simulink model "slewmode"  (R2024a)
settings: Solver=ode45  StartTime=0.0  StopTime=2000  MaxStep=20  RelTol=1e-6  EnableMultiTasking=on
values from neighbouring files (symbols this model uses):
  I = [3000 0 0 ... (first row only)    [Constants_gui.m]    (also in constants.m; mbi.m = [15, .25, .20; set_up_HW7.m = I-Id; setupConstantRateSDA.m)
  invI = inv(I)    [Constants_gui.m]    (also in constants.m; mbi.m; set_up_HW7.m; setupConstantRateSDA.m)
  Kd = 2*zet*wn*I    [Constants_gui.m]    (also in constants.m = 2 * zet * wn * I; mbi.m = -eye(3)*.00002; set_up_HW7.m = 375000; setupConstantRateSDA.m)
  Kp = 2*wn^2*I    [Constants_gui.m]    (also in constants.m = 2 * wn^2 * I; mbi.m = -eye(3)*5.5; set_up_HW7.m = 300000; setupConstantRateSDA.m)
  q_c = q_c / norm(q_c)    [constants.m]
  q_init = q_init/norm(q_init)    [Constants_gui.m]    (also in constants.m = [-0.5 -0.5 -0.5 0.5]; mbi.m = [0 0 0 1]'; set_up_HW7.m = [0 0 0 1]'; setupConstantRateSDA.m)
  wbn_init = pi/30*[0 0 0]'    [Constants_gui.m]    (also in constants.m = pi/180 * [0.1; 0.2; 0.15]; mbi.m = [0 0 0]'; set_up_HW7.m = pi/30*[0 0 .01]'; setupConstantRateSDA.m)
libraries: aerolibutil x2
settings Model: Creator=Mason  LastModifiedBy=robertbergbaum
settings SolverCC: AlgebraicLoopSolver=TrustRegion  MaxZcPerStep=1
settings DataIOCC: LimitDataPoints=on  SaveFormat=Array  SignalLoggingSaveFormat=ModelDataLogs  ReturnWorkspaceOutputs=off
settings OptimizationCC: ExpressionDepthLimit=2147483647  InitFltsAndDblsToZero=on  LifeSpan=inf
settings DebuggingCC: SaveWithParameterizedLinksMsg=none  UnderspecifiedInitializationDetection=Classic  MergeDetectMultiDrivingBlocksExec=none  SignalResolutionControl=TryResolveAllWithWarning  SolverPrmCheckMsg=warning  MultiTaskDSMMsg=warning  MultiTaskCondExecSysMsg=none  FcnCallInpInsideContextMsg=warning  UnconnectedInputMsg=warning  UnconnectedOutputMsg=warning  UnconnectedLineMsg=warning  StateNameClashWarn=warning  SFUnexpectedBacktrackingDiag=warning  SFNoUnconditionalDefaultTransitionDiag=warning  SFExecutionAtInitializationDiag=none  ArithmeticOperatorsInVariantConditions=warning
settings HardwareCC: ProdBitPerPointer=32  ProdBitPerSizeT=32  ProdBitPerPtrDiffT=32  ProdLargestAtomicFloat=None  ProdIntDivRoundTo=Undefined  ProdEndianess=Unspecified  ProdWordSize=32  ProdHWDeviceType=32-bit Generic
settings ModelReferenceCC: EnableRefExpFcnMdlSchedulingChecks=on  PropagateSignalLabelsOutOfModel=off
settings SFSimCC: SimUseLocalCustomCode=off  CustomCodeUndefinedFunction=UseInterfaceOnly
settings RTWCC: RTWUseLocalCustomCode=off  GPUComputeCapability=3.5  DLArmComputeVersion=19.05
settings CodeAppCC: StateflowObjectComments=on
settings GRTTargetCC: TargetFcnLib=ansi_tfl_tmw.mat  TargetLangStandard=C89/C90 (ANSI)  CombineOutputUpdateFcns=off  GRTInterface=on
settings ConfigComp: CovMetricSettings=dw  CovSaveCumulativeToWorkspaceVar=on  CovSaveSingleToWorkspaceVar=on  CovExternalEMLEnable=off

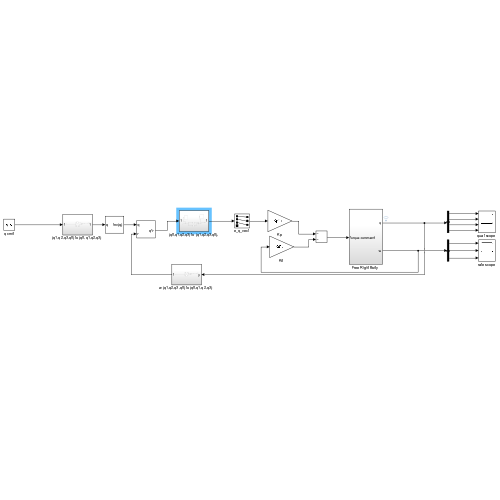
[thumbnail: Simulink's stored preview of the top-level diagram]
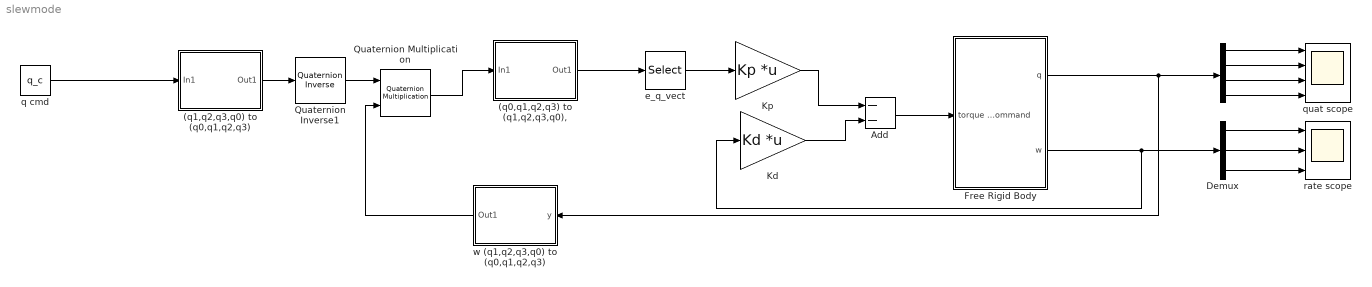
== system slewmode ==
  " " : Demux
      settings: DisplayOption=none
  (q0,q1,q2,q3) to (q1,q2,q3,q0), : Subsystem
  "(q1,q2,q3,q0) to (q0,q1,q2,q3) " : Subsystem
  Add : Sum  Inputs=--
  Demux : Demux  Outputs=3
      settings: DisplayOption=none
  "Free Rigid Body " : Subsystem
  Kd : Gain  Gain=Kd  Multiplication=Matrix(K*u)  SaturateOnIntegerOverflow=on  OutDataTypeStr=Inherit: Same as input  ParamDataTypeStr=Inherit: Same as input
  Kp : Gain  Gain=Kp  Multiplication=Matrix(K*u)  SaturateOnIntegerOverflow=on  OutDataTypeStr=Inherit: Same as input  ParamDataTypeStr=Inherit: Same as input
  Quaternion Inverse1 : aerolibutil/Quaternion Inverse
  Quaternion Multiplication : aerolibutil/Quaternion Multiplication
  e_q_vect : Selector  InputPortWidth=4  IndexOptions=Index vector (dialog)  Indices=[1 2 3]  OutputSizes=1
  q cmd : Constant  Value=q_c  VectorParams1D=off
  quat scope : Scope  NumInputPorts=4
  rate scope : Scope  NumInputPorts=3
  "w (q1,q2,q3,q0) to (q0,q1,q2,q3) " : Subsystem
      settings: PortSchema="{\"entries\":[{\"content\":{\"sides\":[{\"content\":{\"connectorIds\":[\"Out1\"]},\"type\":\"ConnectorPlacement.EquallySpacedRectSide\",\"uuid\":\"97b477ad-5663-4010-b344-d27b8ec095be\"},{\"content\":{\"connectorIds\":[\"In1\"],\"side\":\"RIGHT\"},\"type\":\"ConnectorPlacement.EquallySpacedRectSide\",\"uuid\":\"41fe4029-0263-4427-bdfc-3c26258b8a65\"},{\"content\":{\"side\":\"TOP\"},\"type\":\"ConnectorPlacement.EquallySpacedRectSide\",\"uuid\":\"9fb3a03d-539a-4245-bd7d-8174d3d0797f\"}]},\"type\":\"ConnectorPlacement.EquallySpacedConnector\",\"uuid\":\"44222554-f3ae-4bc6-b92c-7571a5ce84f7\"}],\"packageUris\":[\"http://schema.mathworks.com/mf0/Connector/R2020b\"],\"version\":\"1.0\"}"
  wires:
  Kd/1 -> Add/2
  Demux/2 -> rate scope/2
  Demux/3 -> rate scope/3
  Demux/1 -> rate scope/1
  "Free Rigid Body "/2(w) -> Kd/1, Demux/1
  " "/1 -> quat scope/1
  " "/2 -> quat scope/2
  " "/3 -> quat scope/3
  " "/4 -> quat scope/4
  e_q_vect/1 -> Kp/1
  "Free Rigid Body "/1(q) -> "w (q1,q2,q3,q0) to (q0,q1,q2,q3) "/1(y), " "/1
  Kp/1 -> Add/1
  Add/1 -> "Free Rigid Body "/1(torque command)
  Quaternion Multiplication/1 -> (q0,q1,q2,q3) to (q1,q2,q3,q0),/1(In1)
  (q0,q1,q2,q3) to (q1,q2,q3,q0),/1(Out1) -> e_q_vect/1
  "(q1,q2,q3,q0) to (q0,q1,q2,q3) "/1(Out1) -> Quaternion Inverse1/1
  "w (q1,q2,q3,q0) to (q0,q1,q2,q3) "/1(Out1) -> Quaternion Multiplication/2
  Quaternion Inverse1/1 -> Quaternion Multiplication/1
  q cmd/1 -> "(q1,q2,q3,q0) to (q0,q1,q2,q3) "/1(In1)

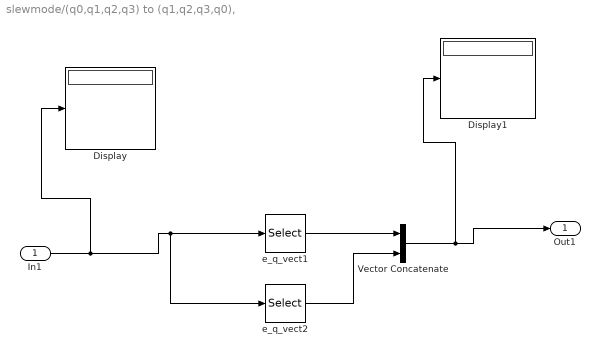
== system slewmode/(q0,q1,q2,q3) to (q1,q2,q3,q0), ==
  In1 : Inport
  Display : Display
  Display1 : Display
  Vector Concatenate : Concatenate
  e_q_vect1 : Selector  InputPortWidth=4  IndexOptions=Index vector (dialog)  Indices=[2 3 4]  OutputSizes=1
  e_q_vect2 : Selector  InputPortWidth=4  IndexOptions=Index vector (dialog)  Indices=[1]  OutputSizes=1
  Out1 : Outport
  wires:
  Vector Concatenate/1 -> Display1/1, Out1/1
  In1/1 -> Display/1, e_q_vect2/1, e_q_vect1/1
  e_q_vect1/1 -> Vector Concatenate/1
  e_q_vect2/1 -> Vector Concatenate/2

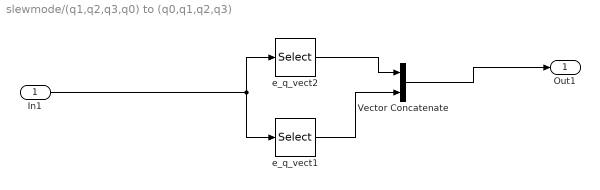
== system slewmode/(q1,q2,q3,q0) to (q0,q1,q2,q3)  ==
  In1 : Inport
  Vector Concatenate : Concatenate
  e_q_vect1 : Selector  InputPortWidth=4  IndexOptions=Index vector (dialog)  Indices=[1 2 3]  OutputSizes=1
  e_q_vect2 : Selector  InputPortWidth=4  IndexOptions=Index vector (dialog)  Indices=[4]  OutputSizes=1
  Out1 : Outport
  wires:
  In1/1 -> e_q_vect2/1, e_q_vect1/1
  e_q_vect2/1 -> Vector Concatenate/1
  e_q_vect1/1 -> Vector Concatenate/2
  Vector Concatenate/1 -> Out1/1

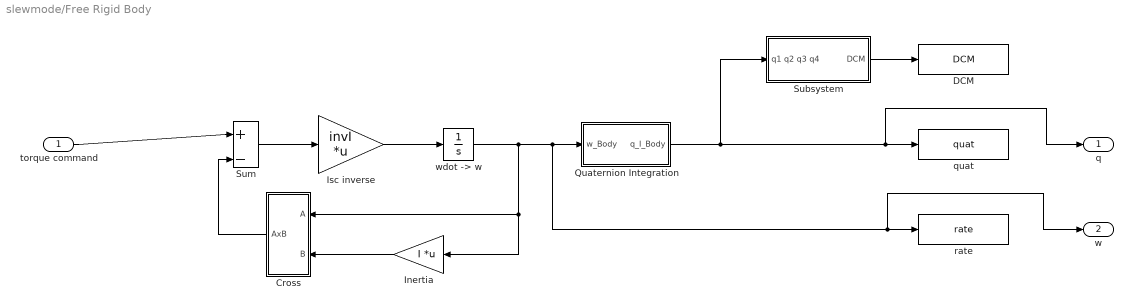
== system slewmode/Free Rigid Body  ==
  torque command : Inport
  Cross : Subsystem
  DCM : ToWorkspace  VariableName=DCM  SaveFormat=Structure With Time  SampleTime=-1
  Inertia : Gain  Gain=I  Multiplication=Matrix(K*u)  SaturateOnIntegerOverflow=on  OutDataTypeStr=Inherit: Same as input  ParamDataTypeStr=Inherit: Same as input
  Isc inverse : Gain  Gain=invI  Multiplication=Matrix(K*u)  SaturateOnIntegerOverflow=on  OutDataTypeStr=Inherit: Same as input  ParamDataTypeStr=Inherit: Same as input
  Quaternion Integration : Subsystem
  Subsystem : Subsystem
  Sum : Sum  Inputs=|+-  InputSameDT=on  SaturateOnIntegerOverflow=on  OutDataTypeStr=Inherit: Same as first input
  quat : ToWorkspace  VariableName=quat  SaveFormat=Structure With Time  SampleTime=-1
  rate : ToWorkspace  VariableName=rate  SaveFormat=Structure With Time  SampleTime=-1
  "wdot -> w" : Integrator  InitialCondition=wbn_init
  q : Outport
  w : Outport  Port=2
  wires:
  Isc inverse/1 -> "wdot -> w"/1
  "wdot -> w"/1 -> w/1, rate/1, Quaternion Integration/1(w_Body), Inertia/1, Cross/1(A)
  Sum/1 -> Isc inverse/1
  torque command/1 -> Sum/1
  Cross/1(AxB) -> Sum/2
  Inertia/1 -> Cross/2(B)
  Quaternion Integration/1(q_I_Body) -> Subsystem/1(q1 q2 q3 q4), q/1, quat/1
  Subsystem/1(DCM) -> DCM/1

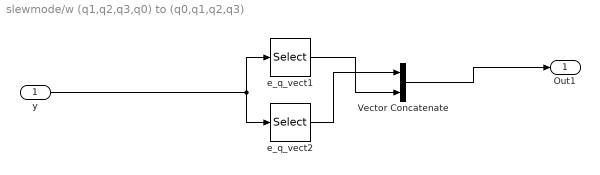
== system slewmode/w (q1,q2,q3,q0) to (q0,q1,q2,q3)  ==
  y : Inport
  Vector Concatenate : Concatenate
  e_q_vect1 : Selector  InputPortWidth=4  IndexOptions=Index vector (dialog)  Indices=[1 2 3]  OutputSizes=1
  e_q_vect2 : Selector  InputPortWidth=4  IndexOptions=Index vector (dialog)  Indices=[4]  OutputSizes=1
  Out1 : Outport
  wires:
  Vector Concatenate/1 -> Out1/1
  e_q_vect1/1 -> Vector Concatenate/2
  e_q_vect2/1 -> Vector Concatenate/1
  y/1 -> e_q_vect1/1, e_q_vect2/1

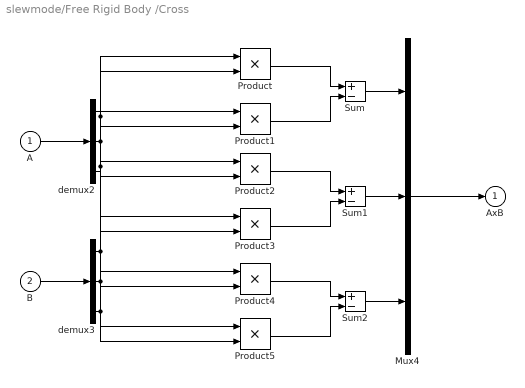
== system slewmode/Free Rigid Body /Cross ==
  A : Inport
  B : Inport  Port=2
  Mux4 : Mux  Inputs=3
  Product{,1..5} (6 alike) : Product  InputSameDT=on  SaturateOnIntegerOverflow=on  OutDataTypeStr=Inherit: Same as first input
  Sum : Sum  Inputs=+-  InputSameDT=on  SaturateOnIntegerOverflow=on  OutDataTypeStr=Inherit: Same as first input
  Sum1 : Sum  Inputs=+-  InputSameDT=on  SaturateOnIntegerOverflow=on  OutDataTypeStr=Inherit: Same as first input
  Sum2 : Sum  Inputs=+-  InputSameDT=on  SaturateOnIntegerOverflow=on  OutDataTypeStr=Inherit: Same as first input
  demux2 : Demux  Outputs=3
      settings: DisplayOption=none
  demux3 : Demux  Outputs=3
      settings: DisplayOption=none
  AxB : Outport  InitialOutput=0
  wires:
  A/1 -> demux2/1
  B/1 -> demux3/1
  demux2/3 -> Product1/1, Product2/1
  demux3/3 -> Product/2, Product3/2
  demux2/1 -> Product3/1, Product4/1
  demux3/2 -> Product1/2, Product4/2
  demux2/2 -> Product/1, Product5/1
  demux3/1 -> Product2/2, Product5/2
  Product/1 -> Sum/1
  Product1/1 -> Sum/2
  Product2/1 -> Sum1/1
  Product3/1 -> Sum1/2
  Product4/1 -> Sum2/1
  Product5/1 -> Sum2/2
  Sum/1 -> Mux4/1
  Sum1/1 -> Mux4/2
  Sum2/1 -> Mux4/3
  Mux4/1 -> AxB/1

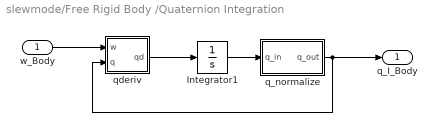
== system slewmode/Free Rigid Body /Quaternion Integration ==
  w_Body : Inport
  Integrator1 : Integrator  InitialCondition=q_init
  q_normalize : Subsystem
  qderiv : Subsystem
  q_I_Body : Outport
  wires:
  w_Body/1 -> qderiv/1(w)
  q_normalize/1(q_out) -> qderiv/2(q), q_I_Body/1
  Integrator1/1 -> q_normalize/1(q_in)
  qderiv/1(qd) -> Integrator1/1

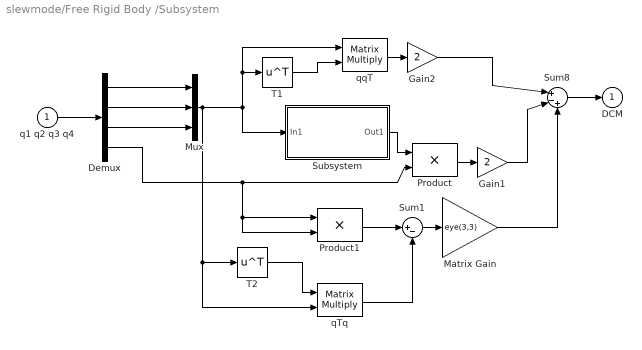
== system slewmode/Free Rigid Body /Subsystem ==
  q1 q2 q3 q4 : Inport
  Demux : Demux
      settings: DisplayOption=none
  Gain1 : Gain  Gain=2  SaturateOnIntegerOverflow=on  OutDataTypeStr=Inherit: Same as input  ParamDataTypeStr=Inherit: Same as input
  Gain2 : Gain  Gain=2  SaturateOnIntegerOverflow=on  OutDataTypeStr=Inherit: Same as input  ParamDataTypeStr=Inherit: Same as input
  Matrix Gain : Gain  Gain=eye(3,3)  SaturateOnIntegerOverflow=on  OutDataTypeStr=Inherit: Same as input  ParamDataTypeStr=Inherit: Same as input
  Mux : Mux  Inputs=3
  Product : Product  InputSameDT=on  SaturateOnIntegerOverflow=on  OutDataTypeStr=Inherit: Same as first input
  Product1 : Product  InputSameDT=on  SaturateOnIntegerOverflow=on  OutDataTypeStr=Inherit: Same as first input
  Subsystem : Subsystem
      mask Display: disp('3x3 cross matrix')
  Sum1 : Sum  Inputs=|+-  InputSameDT=on  SaturateOnIntegerOverflow=on  OutDataTypeStr=Inherit: Same as first input
  Sum8 : Sum  Inputs=|+-+  InputSameDT=on  SaturateOnIntegerOverflow=on  OutDataTypeStr=Inherit: Same as first input
  T1 : Math  Operator=transpose  SignedPower=on
  T2 : Math  Operator=transpose  SignedPower=on
  qTq : Product  Multiplication=Matrix(*)  InputSameDT=on  SaturateOnIntegerOverflow=on  OutDataTypeStr=Inherit: Same as first input
  qqT : Product  Multiplication=Matrix(*)  InputSameDT=on  SaturateOnIntegerOverflow=on  OutDataTypeStr=Inherit: Same as first input
  DCM : Outport  InitialOutput=0
  wires:
  T1/1 -> qqT/2
  Sum8/1 -> DCM/1
  Product/1 -> Gain1/1
  Demux/3 -> Mux/3
  Demux/2 -> Mux/2
  qqT/1 -> Gain2/1
  Gain1/1 -> Sum8/2
  q1 q2 q3 q4/1 -> Demux/1
  Demux/1 -> Mux/1
  Matrix Gain/1 -> Sum8/3
  Product1/1 -> Sum1/1
  qTq/1 -> Sum1/2
  T2/1 -> qTq/1
  Subsystem/1(Out1) -> Product/1
  Mux/1 -> qTq/2, T2/1, qqT/1, T1/1, Subsystem/1(In1)
  Demux/4 -> Product1/2, Product1/1, Product/2
  Sum1/1 -> Matrix Gain/1
  Gain2/1 -> Sum8/1

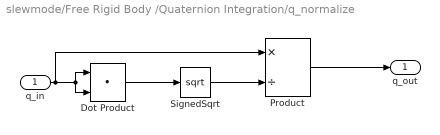
== system slewmode/Free Rigid Body /Quaternion Integration/q_normalize ==
  q_in : Inport  PortDimensions=4
  Dot Product : DotProduct  OutDataTypeStr=Inherit: Inherit via internal rule
  Product : Product  Inputs=*/  InputSameDT=on  SaturateOnIntegerOverflow=on  OutDataTypeStr=Inherit: Same as first input
  SignedSqrt : Sqrt  IntermediateResultsDataTypeStr=double
  q_out : Outport
  wires:
  Product/1 -> q_out/1
  SignedSqrt/1 -> Product/2
  q_in/1 -> Dot Product/2, Dot Product/1, Product/1
  Dot Product/1 -> SignedSqrt/1

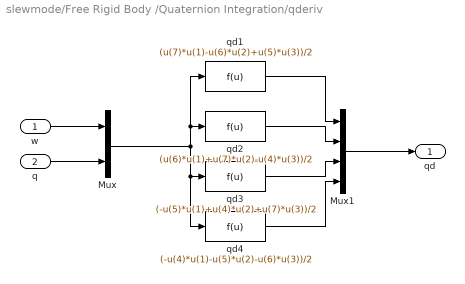
== system slewmode/Free Rigid Body /Quaternion Integration/qderiv ==
  w : Inport
  q : Inport  Port=2
  Mux : Mux  Inputs=2
  Mux1 : Mux
  qd1 : Fcn  Expr=(u(7)*u(1)-u(6)*u(2)+u(5)*u(3))/2
  qd2 : Fcn  Expr=(u(6)*u(1)+u(7)*u(2)-u(4)*u(3))/2
  qd3 : Fcn  Expr=(-u(5)*u(1)+u(4)*u(2)+u(7)*u(3))/2
  qd4 : Fcn  Expr=(-u(4)*u(1)-u(5)*u(2)-u(6)*u(3))/2
  qd : Outport
  wires:
  Mux1/1 -> qd/1
  qd4/1 -> Mux1/4
  qd3/1 -> Mux1/3
  qd2/1 -> Mux1/2
  qd1/1 -> Mux1/1
  Mux/1 -> qd4/1, qd3/1, qd2/1, qd1/1
  q/1 -> Mux/2
  w/1 -> Mux/1

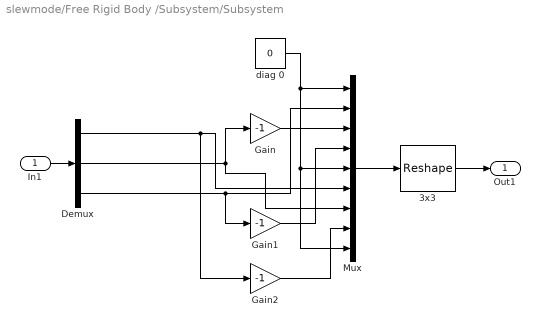
== system slewmode/Free Rigid Body /Subsystem/Subsystem ==
  In1 : Inport
  3x3 : Reshape  OutputDimensionality=Customize  OutputDimensions=[3,3]
  Demux : Demux  Outputs=3
      settings: DisplayOption=none
  Gain : Gain  Gain=-1  SaturateOnIntegerOverflow=on  OutDataTypeStr=Inherit: Same as input  ParamDataTypeStr=Inherit: Same as input
  Gain1 : Gain  Gain=-1  SaturateOnIntegerOverflow=on  OutDataTypeStr=Inherit: Same as input  ParamDataTypeStr=Inherit: Same as input
  Gain2 : Gain  Gain=-1  SaturateOnIntegerOverflow=on  OutDataTypeStr=Inherit: Same as input  ParamDataTypeStr=Inherit: Same as input
  Mux : Mux  Inputs=9
  "diag 0 " : Constant  Value=0
  Out1 : Outport
  wires:
  Gain2/1 -> Mux/8
  Demux/1 -> Gain2/1, Mux/6
  Gain1/1 -> Mux/4
  Demux/2 -> Mux/7, Gain/1
  Gain/1 -> Mux/3
  Demux/3 -> Gain1/1, Mux/2
  Mux/1 -> 3x3/1
  "diag 0 "/1 -> Mux/9, Mux/5, Mux/1
  3x3/1 -> Out1/1
  In1/1 -> Demux/1
